simulink subsystem "Reference_vehicle"  (R2024b)
settings: Solver=VariableStepAuto  StartTime=0.0  StopTime=10.0  RelTol=1e-3
libraries: SignalEditorBlockLib x1
settings Model: Creator=tshintai  LastModifiedBy=tshintai
settings SolverCC: AlgebraicLoopSolver=TrustRegion
settings OptimizationCC: ReuseModelBlockBuffer=off
settings DebuggingCC: UnconnectedInputMsg=warning  UnconnectedOutputMsg=warning  UnconnectedLineMsg=warning
settings ModelReferenceCC: EnableRefExpFcnMdlSchedulingChecks=on
settings RTWCC: GPUComputeCapability=3.5  DLArmComputeVersion=19.05

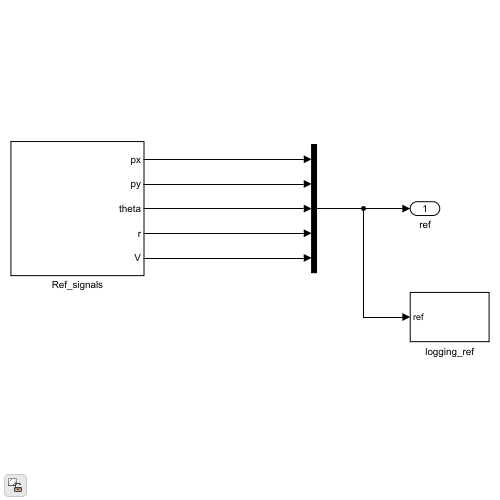
[thumbnail: Simulink's stored preview of the top-level diagram]
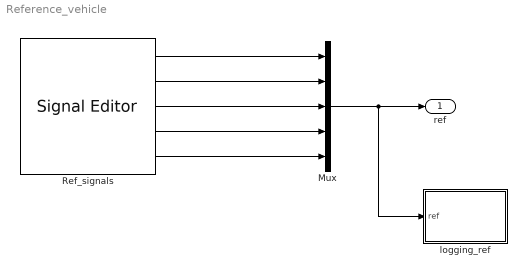
== system Reference_vehicle ==
  Mux : Mux  Inputs=5
  Ref_signals : SignalEditorBlockLib/Signal Editor  FileName=ref_signal_vehicle.mat  ActiveScenario=turn_vehicle  ActiveSignal=py  IsBus=off  OutputBusObjectStr=Bus: BusObject  SampleTime=0  ZeroCross=off  OutputAfterFinalValue=Extrapolation  Unit=inherit  PreserveSignalName=on  ApplySigPropsToAllScenarios=on  ApplySigPropsToAllSignals=off
  logging_ref : Subsystem
  ref : Outport
  wires:
  Mux/1 -> ref/1, logging_ref/1(ref)
  Ref_signals/1 -> Mux/1
  Ref_signals/2 -> Mux/2
  Ref_signals/3 -> Mux/3
  Ref_signals/4 -> Mux/4
  Ref_signals/5 -> Mux/5

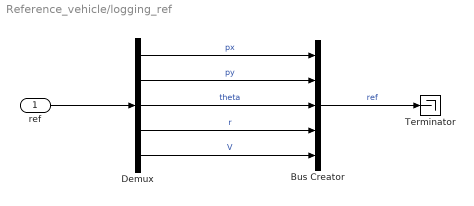
== system Reference_vehicle/logging_ref ==
  ref : Inport
  Bus Creator : BusCreator  Inputs=5
  Demux : Demux  Outputs=5
  Terminator : Terminator
  wires:
  Demux/1 -> Bus Creator/1  "px"
  ref/1 -> Demux/1
  Demux/4 -> Bus Creator/4  "r"
  Demux/2 -> Bus Creator/2  "py"
  Bus Creator/1 -> Terminator/1  "ref"
  Demux/5 -> Bus Creator/5  "V"
  Demux/3 -> Bus Creator/3  "theta"
